simulink model "CDR_240702"  (R2019b)
settings: Solver=ode4  StartTime=0.0  StopTime=inf  FixedStep=BKIN_STEP_TIME  RelTol=1e-3  EnableMultiTasking=on
StartFcn:
  |  warndlg('Dexterit-E models cannot run under simulation. Please compile your model and run it from within Dexterit-E.');set_param(bdroot,'SimulationCommand','stop')
model workspace (MAT data in the model file):
  BKIN_KINEMATIC_FRAME_SIZE = 400
  BKIN_STEP_TIME = 0.00025
  COHERENCY = 9
  CONST_A = 1
  CONST_B = 2
  CONST_C = 3
  CONST_D = 4
  DIRECTION = 10
  DOT_AREA_RADIUS = 5
  DOT_DELAY = 4
  DOT_TARGET = 7
  D_REACH_TARG = 4
  D_START_TARG = 2
  E_DOT_ON = 3
  E_D_REACHED = 5
  E_ND_REACHED = 4
  E_NO_EVENT = 0
  E_REACH_ON = 2
  E_START_ON = 1
  E_TIMED_OUT = 7
  E_TOO_SLOW = 6
  E_TRIAL_END = 8
  HEIGHT = 5
  INCREMENT_TRIGGER = 12
  INC_RES = 7
  INIT_COLOR = 7
  LABEL_HEIGHT = 10
  LABEL_TEXT = 9
  LENGTH = 4
  LOAD_1 = 8
  MAX_REACH_TIME = 1
  ND_REACH_TARG = 3
  ND_START_TARG = 1
  NUMBER_OF_DOTS = 6
  PUSH_BACK = 9
  RADIUS_VIS = 3
  RAMP_DURATION = 10
  RESCALE = 8
  SPEED = 11
  STROKE_COLOR = 8
  STROKE_WIDTH = 6
  TIME_OUT = 2
  TIME_OUT_LABEL = 6
  TOO_SLOW_LABEL = 5
  TRIAL_DELAY = 3
  col_x = 1
  col_y = 2
undefined symbols (not defined in the file): slselsubs
libraries: Video x8, KINARM_EP_loads x5, General x3, KINARM_general x3, slrtlib x2
settings Model: ModifiedComment=chris -- Wed Feb 16 09:18:30 2005 -- Version 1.1384  ModifiedHistory=Feb 16/05 - Add error repeat, add offset ramp  ExtModeArmWhenConnect=off  ExtModeLogAll=off  OrderedModelArguments=off  Creator=Chris Grebeldinger  LastModifiedBy=User
settings SolverCC: AutoInsertRateTranBlk=on
settings DataIOCC: SaveFormat=Array  SignalLoggingSaveFormat=ModelDataLogs  SaveOutput=off  SaveTime=off  ReturnWorkspaceOutputs=off  SignalLoggingName=sigsOut
settings OptimizationCC: BlockReduction=off  BooleanDataType=off  OptimizeBlockIOStorage=off  BufferReuse=off  GlobalBufferReuse=off  ExpressionFolding=off  ExpressionDepthLimit=2147483647  LocalBlockOutputs=off  InitFltsAndDblsToZero=on  LifeSpan=inf  OptimizeDataStoreBuffers=off  BusAssignmentInplaceUpdate=off
settings DebuggingCC: SaveWithParameterizedLinksMsg=none  UnderspecifiedInitializationDetection=Classic  MergeDetectMultiDrivingBlocksExec=none  SignalResolutionControl=TryResolveAllWithWarning  MultiTaskDSMMsg=warning  FcnCallInpInsideContextMsg=warning  BusObjectLabelMismatch=none  StateNameClashWarn=warning  StrictBusMsg=ErrorOnBusTreatedAsVector  SFUnexpectedBacktrackingDiag=warning  SFNoUnconditionalDefaultTransitionDiag=warning  SFExecutionAtInitializationDiag=none  ArithmeticOperatorsInVariantConditions=warning
settings HardwareCC: ProdBitPerPointer=32  ProdBitPerSizeT=32  ProdBitPerPtrDiffT=32  ProdLargestAtomicFloat=None  ProdWordSize=32  ProdLongLongMode=on  ProdHWDeviceType=Generic->32-bit x86 compatible  TargetHWDeviceType=32-bit Generic
settings ModelReferenceCC: PropagateSignalLabelsOutOfModel=off
settings SFSimCC: SimCustomHeaderCode="#include \"stdlib.h\""  SFSimEcho=off  SimUseLocalCustomCode=off  SimParseCustomCode=off  CustomCodeUndefinedFunction=UseInterfaceOnly
settings RTWCC: Description=Simulink Real-Time  SystemTargetFile=slrt.tlc  TemplateMakefile=slrt_default_tmf  RTWUseLocalCustomCode=off  CustomSourceCode="#include \"stdlib.h\""  CodeExecutionProfiling=on  RTWCompilerOptimization=on
settings CodeAppCC: MaxIdLength=63  StateflowObjectComments=on
settings SimulinkRealTimeCC: TargetFcnLib=ansi_tfl_tmw.mat  GeneratePreprocessorConditionals=Disable all  PreserveStateflowLocalDataDimensions=off
settings ConfigComp: CovMetricSettings=dw  CovHtmlReporting=on  CovSaveCumulativeToWorkspaceVar=on  CovSaveSingleToWorkspaceVar=on  CovExternalEMLEnable=off

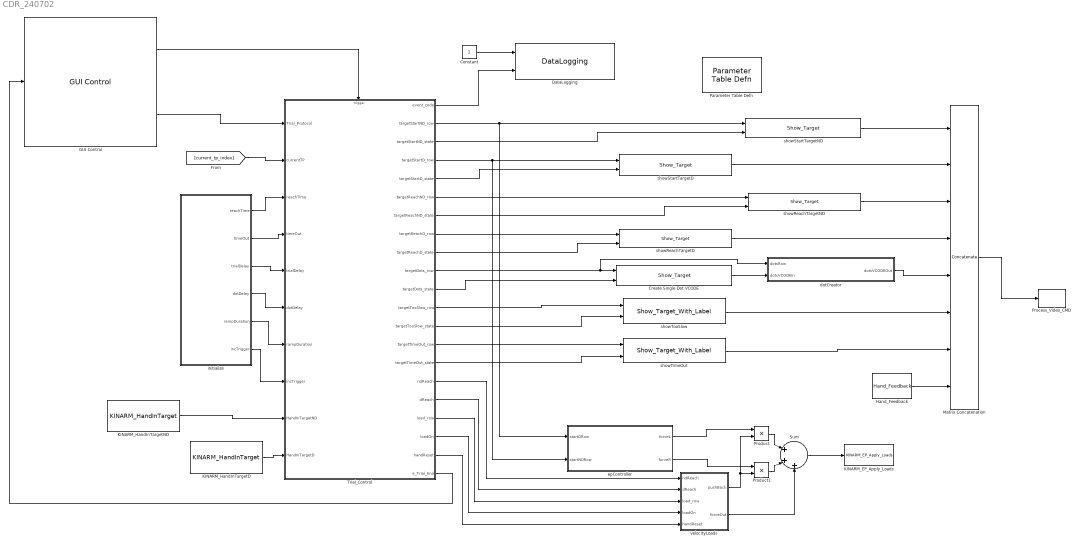
== system CDR_240702 ==
  Constant : Constant
  Create Single Dot VCODE : Video/Show_Target  target_type=Circle  num_states=1  attribcol1=[INIT_COLOR 0 0 RADIUS_VIS]  attribcol2=[0 0 0 0]  attribcol3=[0 0 0 0]  attribcol4=[0 0 0 0]  attribcol5=[0 0 0 0]  stateindices_padding=[0 0 0 0 0 0 0;0 0 0 0 0 0 0;0 0 0 0 0 0 0;0 0 0 0 0 0 0;0 0 0 0 0 0 0]  source=dialog  opacity=100  target_display=Both subject and operator displays  num_col=4
  DataLogging : General/DataLogging  log_event_codes=on  log_analog_inputs=off  show_time_remaining=off  ecat_include=on
  GUI Control : General/GUI Control  task_version=1.0  show_repeat_trial_flag=off  use_custom_tp=off  target_type_str=Circle  Target_Type=1  XYcols=[1 2]  Vcols=3  Lcols=4  indices_padding=[0 0 0 0;0 0 0 0]  target_table_rows=64  load_table_rows=20  tp_table_rows=100
  Hand_Feedback : KINARM_general/Hand_Feedback  feedback_cntl_src=none
  KINARM_EP_Apply_Loads : KINARM_EP_loads/KINARM_EP_Apply_Loads  up_duration=100  down_duration=100  max_force=15
  KINARM_HandInTargetD : KINARM_general/KINARM_HandInTarget  use_dominant_hand=on  target_type=Rectangle  num_states=1  attribcol1=[ LENGTH HEIGHT 0]  attribcol2=[0 0 0]  attribcol3=[0 0 0]  attribcol4=[0 0 0]  attribcol5=[0 0 0]
  KINARM_HandInTargetND : KINARM_general/KINARM_HandInTarget  use_dominant_hand=off  target_type=Rectangle  num_states=1  attribcol1=[ LENGTH HEIGHT 0]  attribcol2=[0 0 0]  attribcol3=[0 0 0]  attribcol4=[0 0 0]  attribcol5=[0 0 0]
  Matrix Concatenation : Concatenate  NumInputs=8  Mode=Multidimensional array
  Parameter Table Defn : General/Parameter Table Defn  ShowInLibBrowser=0
  Process_Video_CMD : Video/Process_Video_CMD  video_delay=0
  Product : Product
  Product1 : Product
  Sum : Sum  Inputs=|+++
  Trial_Control : Stateflow chart  TreatAsAtomicUnit=on
  dotCreator : Subsystem
  epController : Subsystem
  initialize : Subsystem
  showReachTargetD : Video/Show_Target  target_type=Rectangle  num_states=1  attribcol1=[INIT_COLOR STROKE_COLOR STROKE_WIDTH LENGTH HEIGHT 0]  attribcol2=[0 0 0 0 0 0]  attribcol3=[0 0 0 0 0 0]  attribcol4=[0 0 0 0 0 0]  attribcol5=[0 0 0 0 0 0]  stateindices_padding=[0 0 0 0 0;0 0 0 0 0;0 0 0 0 0;0 0 0 0 0;0 0 0 0 0]  source=dialog  opacity=100  target_display=Both subject and operator displays  num_col=6
  showReachTargetND : Video/Show_Target  target_type=Rectangle  num_states=1  attribcol1=[INIT_COLOR STROKE_COLOR STROKE_WIDTH LENGTH HEIGHT 0]  attribcol2=[0 0 0 0 0 0]  attribcol3=[0 0 0 0 0 0]  attribcol4=[0 0 0 0 0 0]  attribcol5=[0 0 0 0 0 0]  stateindices_padding=[0 0 0 0 0;0 0 0 0 0;0 0 0 0 0;0 0 0 0 0;0 0 0 0 0]  source=dialog  opacity=100  target_display=Both subject and operator displays  num_col=6
  showStartTargetD : Video/Show_Target  target_type=Rectangle  num_states=1  attribcol1=[INIT_COLOR STROKE_COLOR STROKE_WIDTH LENGTH HEIGHT 0]  attribcol2=[0 0 0 0 0 0]  attribcol3=[0 0 0 0 0 0]  attribcol4=[0 0 0 0 0 0]  attribcol5=[0 0 0 0 0 0]  stateindices_padding=[0 0 0 0 0;0 0 0 0 0;0 0 0 0 0;0 0 0 0 0;0 0 0 0 0]  source=dialog  opacity=100  target_display=Both subject and operator displays  num_col=6
  showStartTargetND : Video/Show_Target  target_type=Rectangle  num_states=1  attribcol1=[INIT_COLOR STROKE_COLOR STROKE_WIDTH LENGTH HEIGHT 0]  attribcol2=[0 0 0 0 0 0]  attribcol3=[0 0 0 0 0 0]  attribcol4=[0 0 0 0 0 0]  attribcol5=[0 0 0 0 0 0]  stateindices_padding=[0 0 0 0 0;0 0 0 0 0;0 0 0 0 0;0 0 0 0 0;0 0 0 0 0]  source=dialog  opacity=100  target_display=Both subject and operator displays  num_col=6
  showTimeOut : Video/Show_Target_With_Label  target_type=Circle  num_states=1  attribcol1=[0 0 0 0 LABEL_TEXT INIT_COLOR LABEL_HEIGHT]  attribcol2=[0 0 0 0 0 0 0]  attribcol3=[0 0 0 0 0 0 0]  attribcol4=[0 0 0 0 0 0 0]  attribcol5=[0 0 0 0 0 0 0]  stateindices_padding=[0 0 0 0;0 0 0 0;0 0 0 0;0 0 0 0;0 0 0 0]  source=dialog  opacity=100  target_display=Both subject and operator displays
  showTooSlow : Video/Show_Target_With_Label  target_type=Circle  num_states=1  attribcol1=[0 0 0 0 LABEL_TEXT INIT_COLOR LABEL_HEIGHT]  attribcol2=[0 0 0 0 0 0 0]  attribcol3=[0 0 0 0 0 0 0]  attribcol4=[0 0 0 0 0 0 0]  attribcol5=[0 0 0 0 0 0 0]  stateindices_padding=[0 0 0 0;0 0 0 0;0 0 0 0;0 0 0 0;0 0 0 0]  source=dialog  opacity=100  target_display=Both subject and operator displays
  velocityLoads : Subsystem
  wires:
  KINARM_HandInTargetND/1 -> Trial_Control/9(HandInTargetND)
  GUI Control/2 -> Trial_Control/1(Trial_Protocol)
  Trial_Control/21(e_Trial_End) -> GUI Control/1
  GUI Control/1 -> Trial_Control/Trigger
  Trial_Control/7(targetReachND_state) -> showReachTargetND/2
  Trial_Control/6(targetReachND_row) -> showReachTargetND/1
  Matrix Concatenation/1 -> Process_Video_CMD/1
  Hand_Feedback/1 -> Matrix Concatenation/8
  Trial_Control/8(targetReachD_row) -> showReachTargetD/1
  Trial_Control/9(targetReachD_state) -> showReachTargetD/2
  Trial_Control/1(event_code) -> DataLogging/2
  Constant/1 -> DataLogging/1
  KINARM_HandInTargetD/1 -> Trial_Control/10(HandInTargetD)
  initialize/1(reachTime) -> Trial_Control/3(reachTime)
  initialize/2(timeOut) -> Trial_Control/4(timeOut)
  Trial_Control/11(targetDots_state) -> Create Single Dot VCODE/2
  Create Single Dot VCODE/1 -> dotCreator/2(dotsVCODEIn)
  Trial_Control/10(targetDots_row) -> dotCreator/1(dotsRow), Create Single Dot VCODE/1
  dotCreator/1(dotsVCODEOut) -> Matrix Concatenation/5
  showReachTargetND/1 -> Matrix Concatenation/3
  showReachTargetD/1 -> Matrix Concatenation/4
  showStartTargetD/1 -> Matrix Concatenation/2
  showStartTargetND/1 -> Matrix Concatenation/1
  initialize/3(trialDelay) -> Trial_Control/5(trialDelay)
  Trial_Control/2(targetStartND_row) -> epController/1(startDRow), showStartTargetND/1
  Trial_Control/5(targetStartD_state) -> showStartTargetD/2
  initialize/4(dotDelay) -> Trial_Control/6(dotDelay)
  [current_tp_index] -> Trial_Control/2(currentTP)
  Trial_Control/3(targetStartND_state) -> showStartTargetND/2
  Trial_Control/4(targetStartD_row) -> showStartTargetD/1, epController/2(startNDRow)
  Trial_Control/18(load_row) -> velocityLoads/3(load_row)
  Trial_Control/16(ndReach) -> velocityLoads/1(ndReach)
  Trial_Control/17(dReach) -> velocityLoads/2(dReach)
  Trial_Control/19(loadOn) -> velocityLoads/4(loadOn)
  Sum/1 -> KINARM_EP_Apply_Loads/1
  velocityLoads/2(forceOut) -> Sum/3
  Product1/1 -> Sum/2
  Product/1 -> Sum/1
  Trial_Control/20(handReset) -> velocityLoads/5(handReset)
  epController/1(forceL) -> Product/1
  epController/2(forceR) -> Product1/1
  initialize/6(incTrigger) -> Trial_Control/8(incTrigger)
  Trial_Control/12(targetTooSlow_row) -> showTooSlow/1
  Trial_Control/13(targetTooSlow_state) -> showTooSlow/2
  Trial_Control/15(targetTimeOut_state) -> showTimeOut/2
  Trial_Control/14(targetTimeOut_row) -> showTimeOut/1
  showTimeOut/1 -> Matrix Concatenation/7
  showTooSlow/1 -> Matrix Concatenation/6
  velocityLoads/1(pushBack) -> Product/2, Product1/2
  initialize/5(rampDuration) -> Trial_Control/7(rampDuration)

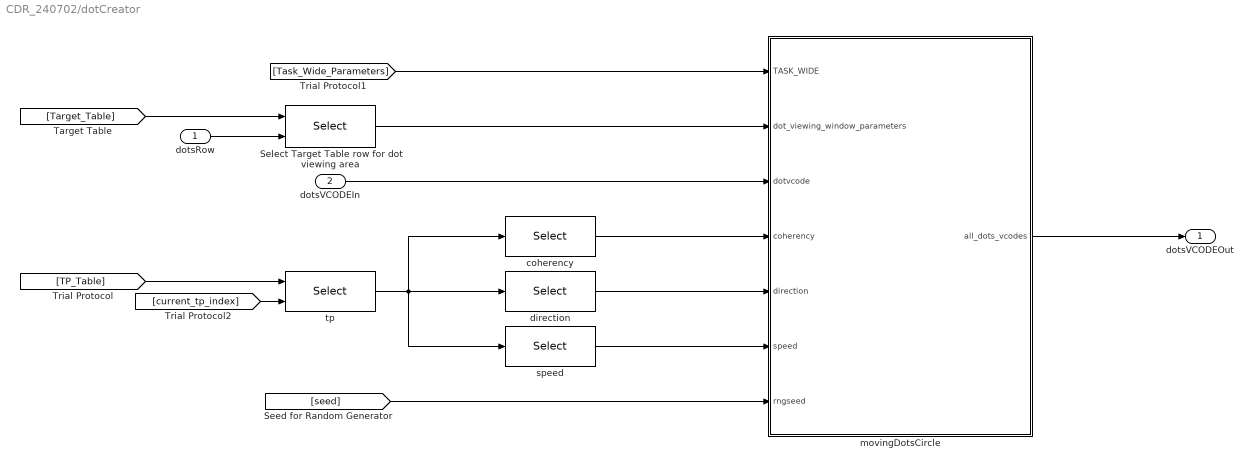
== system CDR_240702/dotCreator ==
  dotsRow : Inport
  dotsVCODEIn : Inport  Port=2
  Select Target Table row for dot viewing area : Selector  NumberOfDimensions=2  IndexOptions=Index vector (port),Index vector (dialog)  Indices=[SPEED],[col_x col_y]  OutputSizes=1,1
  coherency : Selector  IndexOptions=Index vector (dialog)  Indices=[COHERENCY]  OutputSizes=1
  direction : Selector  IndexOptions=Index vector (dialog)  Indices=[DIRECTION]  OutputSizes=1
  movingDotsCircle : MATLAB Function  TreatAsAtomicUnit=on  SystemSampleTime=0.02
  speed : Selector  IndexOptions=Index vector (dialog)  Indices=[SPEED]  OutputSizes=1
  tp : Selector  NumberOfDimensions=2  IndexOptions=Index vector (port),Select all  Indices=[COHERENCY],100  OutputSizes=1,100
  dotsVCODEOut : Outport
  wires:
  movingDotsCircle/1(all_dots_vcodes) -> dotsVCODEOut/1
  Select Target Table row for dot viewing area/1 -> movingDotsCircle/2(dot_viewing_window_parameters)
  coherency/1 -> movingDotsCircle/4(coherency)
  direction/1 -> movingDotsCircle/5(direction)
  speed/1 -> movingDotsCircle/6(speed)
  [seed] -> movingDotsCircle/7(rngseed)
  [Target_Table] -> Select Target Table row for dot viewing area/1
  dotsVCODEIn/1 -> movingDotsCircle/3(dotvcode)
  dotsRow/1 -> Select Target Table row for dot viewing area/2
  [Task_Wide_Parameters] -> movingDotsCircle/1(TASK_WIDE)
  [TP_Table] -> tp/1
  [current_tp_index] -> tp/2
  tp/1 -> direction/1, speed/1, coherency/1

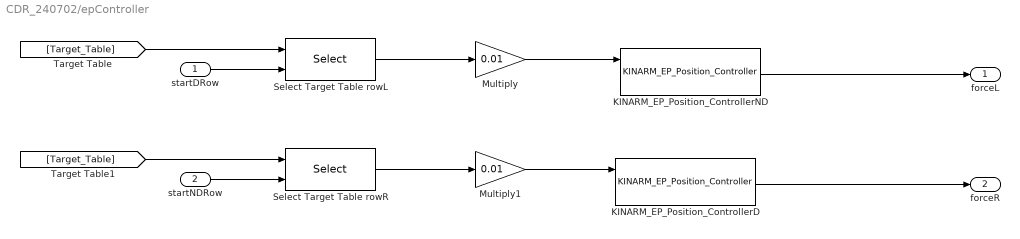
== system CDR_240702/epController ==
  startDRow : Inport
  startNDRow : Inport  Port=2
  KINARM_EP_Position_ControllerD : KINARM_EP_loads/KINARM_EP_Position_Controller  use_dom_hand=on  inertias_for_FF=KINARM End Point robot  gain_choice=Standard Movement  sample_time=0.001
  KINARM_EP_Position_ControllerND : KINARM_EP_loads/KINARM_EP_Position_Controller  use_dom_hand=off  inertias_for_FF=KINARM End Point robot  gain_choice=Standard Movement  sample_time=0.001
  Multiply : Gain  Gain=0.01
  Multiply1 : Gain  Gain=0.01
  Select Target Table rowL : Selector  NumberOfDimensions=2  IndexOptions=Index vector (port),Index vector (dialog)  Indices=[SPEED],[col_x col_y]  OutputSizes=1,1
  Select Target Table rowR : Selector  NumberOfDimensions=2  IndexOptions=Index vector (port),Index vector (dialog)  Indices=[SPEED],[col_x col_y]  OutputSizes=1,1
  forceL : Outport
  forceR : Outport  Port=2
  wires:
  [Target_Table] -> Select Target Table rowL/1
  startDRow/1 -> Select Target Table rowL/2
  startNDRow/1 -> Select Target Table rowR/2
  [Target_Table] -> Select Target Table rowR/1
  Select Target Table rowR/1 -> Multiply1/1
  KINARM_EP_Position_ControllerND/1 -> forceL/1
  Select Target Table rowL/1 -> Multiply/1
  Multiply/1 -> KINARM_EP_Position_ControllerND/1
  Multiply1/1 -> KINARM_EP_Position_ControllerD/1
  KINARM_EP_Position_ControllerD/1 -> forceR/1

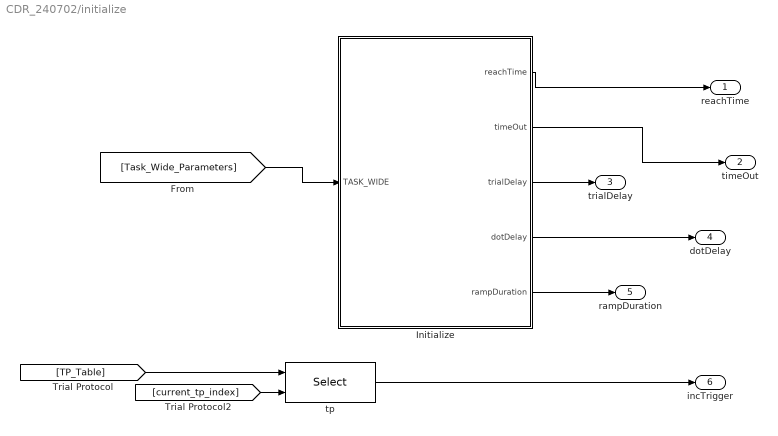
== system CDR_240702/initialize ==
  Initialize : MATLAB Function  TreatAsAtomicUnit=on
  tp : Selector  NumberOfDimensions=2  IndexOptions=Index vector (port),Index vector (dialog)  Indices=[COHERENCY],[INCREMENT_TRIGGER]  OutputSizes=1,100
  reachTime : Outport
  timeOut : Outport  Port=2
  trialDelay : Outport  Port=3
  dotDelay : Outport  Port=4
  rampDuration : Outport  Port=5
  incTrigger : Outport  Port=6
  wires:
  Initialize/1(reachTime) -> reachTime/1
  [Task_Wide_Parameters] -> Initialize/1(TASK_WIDE)
  Initialize/2(timeOut) -> timeOut/1
  Initialize/3(trialDelay) -> trialDelay/1
  Initialize/4(dotDelay) -> dotDelay/1
  tp/1 -> incTrigger/1
  [current_tp_index] -> tp/2
  [TP_Table] -> tp/1
  Initialize/5(rampDuration) -> rampDuration/1

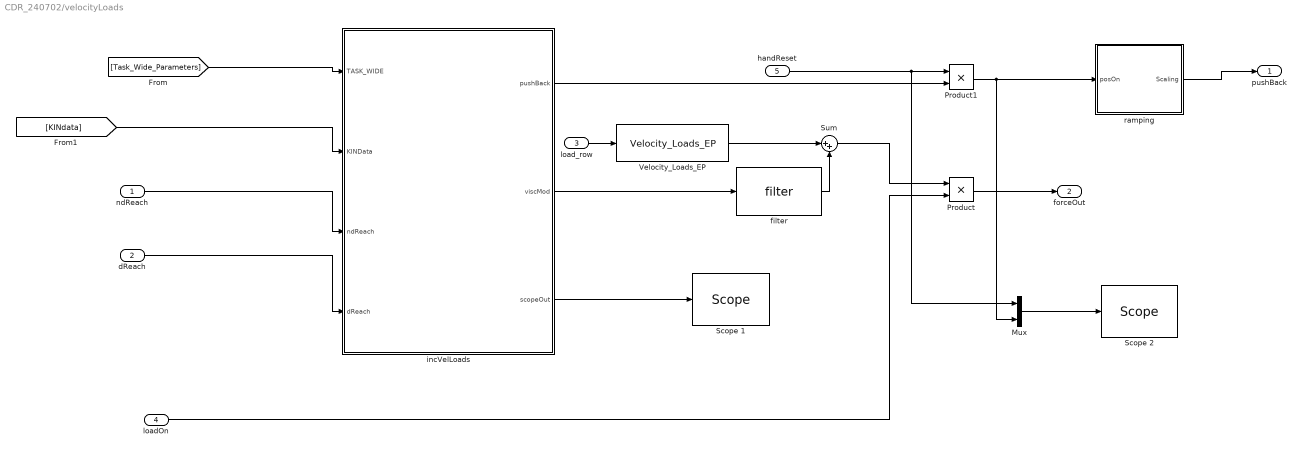
== system CDR_240702/velocityLoads ==
  ndReach : Inport
  dReach : Inport  Port=2
  load_row : Inport  Port=3
  loadOn : Inport  Port=4
  handReset : Inport  Port=5
  Mux : Mux  Inputs=2
  Product : Product
  Product1 : Product
  Scope 1 : slrtlib/Displays and Logging/Scope   scopeno=1  scopetype=Target  autostart=on  viewmode=Numerical  formatstr='%15.6f'  grid=on  ylimits=[0,0]  nosamples=250  noprepostsamples=0  interleave=1  triggermode=FreeRun  triggersignal=1  trigsignalfromport=off  triggerlevel=0.0  triggerslope=Either  triggerscope=1  triggersample=0  filename=data.dat  mode=Lazy  writesize=512  autorestart=off  dynamicfilemode=off  maxwritefilesize=512*1024^2
  Scope 2 : slrtlib/Displays and Logging/Scope   scopeno=2  scopetype=Target  autostart=on  viewmode=Numerical  formatstr='%15.6f'  grid=on  ylimits=[0,0]  nosamples=250  noprepostsamples=0  interleave=1  triggermode=FreeRun  triggersignal=1  trigsignalfromport=off  triggerlevel=0.0  triggerslope=Either  triggerscope=1  triggersample=0  filename=data.dat  mode=Lazy  writesize=512  autorestart=off  dynamicfilemode=off  maxwritefilesize=512*1024^2
  Sum : Sum  Inputs=|++
  Velocity_Loads_EP : KINARM_EP_loads/Velocity_Loads_EP  use_dom_hand=on  loadcol=[1 2 3 4]  source=dialog  scaling=1  stability=on
  filter : KINARM_EP_loads/Velocity_Loads_EP/filter  SystemSampleTime=-1  Latency=0  AutoFrameSizeCalculation=off
  incVelLoads : MATLAB Function  TreatAsAtomicUnit=on  SystemSampleTime=0.02
  ramping : Subsystem  mask(Perturbation){}
  pushBack : Outport
  forceOut : Outport  Port=2
  wires:
  [Task_Wide_Parameters] -> incVelLoads/1(TASK_WIDE)
  incVelLoads/2(viscMod) -> filter/1
  Product/1 -> forceOut/1
  loadOn/1 -> Product/2
  load_row/1 -> Velocity_Loads_EP/1
  ndReach/1 -> incVelLoads/3(ndReach)
  dReach/1 -> incVelLoads/4(dReach)
  Velocity_Loads_EP/1 -> Sum/1
  incVelLoads/3(scopeOut) -> Scope 1/1
  incVelLoads/1(pushBack) -> Product1/2
  handReset/1 -> Mux/1, Product1/1
  Product1/1 -> ramping/1(posOn), Mux/2
  [KINdata] -> incVelLoads/2(KINData)
  Sum/1 -> Product/1
  filter/1 -> Sum/2
  Mux/1 -> Scope 2/1
  ramping/1(Scaling) -> pushBack/1

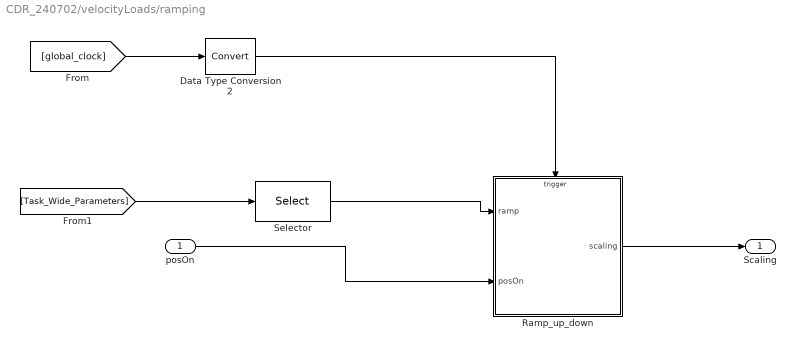
== system CDR_240702/velocityLoads/ramping ==
  posOn : Inport
  Data Type Conversion2 : DataTypeConversion
  Ramp_up_down : Stateflow chart  TreatAsAtomicUnit=on
  Selector : Selector  NumberOfDimensions=2  InputPortWidth=3  IndexOptions=Index vector (dialog),Select all  Indices=[RAMP_DURATION],[3]  OutputSizes=slselsubs([(-2),(-2)],1),1
  Scaling : Outport
  wires:
  Ramp_up_down/1(scaling) -> Scaling/1
  [global_clock] -> Data Type Conversion2/1
  Data Type Conversion2/1 -> Ramp_up_down/Trigger
  [Task_Wide_Parameters] -> Selector/1
  Selector/1 -> Ramp_up_down/1(ramp)
  posOn/1 -> Ramp_up_down/2(posOn)

== stateflow chart CDR_240702/Trial_Control ==
  settings: sampleTime=0.001
  state MainTrial
    state showReach/
      entry:
      event_code = E_REACH_ON;
      targetReachND_state = 1;
      targetReachD_state = 1;
    state showStartTargets/
      entry:
      event_code = E_START_ON;
      targetStartND_state = 1;
      targetStartD_state = 1;
      handReset = 0;
      loadOn = 0;
    state showDots/
      entry:
      loadOn = 1;
      event_code = E_DOT_ON;
      targetDots_state = 1;
    state leftReached/
      entry:
      event_code = E_D_REACHED;
      dReach = dReach + 1;
    state rightReached/
      entry:
      event_code = E_ND_REACHED;
      ndReach = ndReach + 1;
    state noIncrement/
      entry:
      ndReach = 0;
      dReach = 0;
    state tooSlow/
      % Set the post-trial delay.
      entry:
      event_code = E_TOO_SLOW;
      targetTooSlow_state = 1;
      targetDots_state = 0;
    state timedOut/
      % Set the post-trial delay.
      entry:
      event_code = E_TIMED_OUT;
      targetTimeOut_state = 1;
      targetDots_state = 0;
    state statesOff/
      entry:
      targetDots_state = 0;
      targetReachND_state = 0;
      targetReachD_state = 0;
      targetStartND_state = 0;
      targetStartD_state = 0;
      loadOn = 0;
      handReset = 1;
    state EndOfTrial/
      % Set the post-trial delay.
      entry:
      targetTooSlow_state = 0;
      targetTimeOut_state = 0;
      event_code = E_TRIAL_END;
    showStartTargets -> timedOut [order 2] : after(timeOut, msec)
    showStartTargets -> showReach [order 1] : [HandInTargetD(targetStartD_row) == 1 && HandInTargetND(targetStartND_row) == 1]
    showReach -> showStartTargets [order 1] : [HandInTargetD(targetStartD_row) == 0]
    showReach -> showStartTargets [order 2] : [HandInTargetND(targetStartND_row) == 0]
    showReach -> showDots [order 3] : after(dotDelay,msec)
    showDots -> leftReached [order 3] : [HandInTargetD(targetReachD_row) == 1]
    showDots -> rightReached [order 2] : [HandInTargetND(targetReachND_row) == 1]
    leftReached -> (junction 76)
    showDots -> tooSlow [order 1] : after(reachTime, msec)
    rightReached -> (junction 76)
    (junction 76) -> noIncrement [order 2] : [incTrigger == 0]
    (junction 76) -> statesOff [order 1] : after(trialDelay, msec)
    noIncrement -> statesOff : after(trialDelay, msec)
    tooSlow -> EndOfTrial : after(trialDelay*4,msec)
    timedOut -> EndOfTrial : after(trialDelay*4,msec)
    statesOff -> EndOfTrial : after(rampDuration, msec)
  state Initialize/
    entry:
    targetDots_row = Trial_Protocol(DOT_TARGET);
    load_row = Trial_Protocol(LOAD_1);
    targetDots_state = 0;
    targetStartND_row = Trial_Protocol(ND_START_TARG);
    targetStartND_state = 0;
    targetStartD_row = Trial_Protocol(D_START_TARG);
    targetStartD_state = 0;
    targetReachND_row = Trial_Protocol(ND_REACH_TARG);
    targetReachND_state = 0;
    targetReachD_row = Trial_Protocol(D_REACH_TARG);
    targetReachD_state = 0;
    targetTooSlow_row = Trial_Protocol(TOO_SLOW_LABEL);
    targetTooSlow_state = 0;
    targetTimeOut_row = Trial_Protocol(TIME_OUT_LABEL);
    targetTimeOut_state = 0;
    ndReach = 0;
    dReach = 0;
  state Inter_Trial_State/
    entry:
    event_code = 0;
    targetDots_state = 0;
    targetReachND_state = 0;
    targetReachD_state = 0;
    targetStartND_state = 0;
    targetStartD_state = 0;
    targetTooSlow_state = 0;
    targetTimeOut_state = 0;
    handReset = 0;
    loadOn = 0;
    e_Trial_End;
  (default) -> Initialize
  Initialize -> showStartTargets : [currentTP > 0]
  Inter_Trial_State -> showStartTargets : after(1, msec)
  MainTrial -> Inter_Trial_State : e_ExitTrialNow
  EndOfTrial -> Inter_Trial_State : after(rampDuration*2,msec)
  data: Trial_Protocol input double; currentTP input; event_code output [0..] =0; targetStartND_row output; targetStartND_state output; targetStartD_row output; targetStartD_state output; targetReachND_row output [1..32]; targetReachND_state output double; targetReachD_row output double; targetReachD_state output double; targetDots_row output; targetDots_state output; targetTooSlow_row output; targetTooSlow_state output; targetTimeOut_row output; targetTimeOut_state output; reachTime input; timeOut input; trialDelay input; dotDelay input; rampDuration input; incTrigger input; HandInTargetND input double; HandInTargetD input; ndReach output; dReach output; load_row output; loadOn output; handReset output
  data targetReachND_row settings: description=index of the row currently being used in the TargetTable
  events: e_clk input RISING_EDGE_EVENT; e_ExitTrialNow input EITHER_EDGE_EVENT; e_Trial_End output EITHER_EDGE_EVENT

== matlab function CDR_240702/dotCreator/movingDotsCircle ==
  data: TASK_WIDE input; dot_viewing_window_parameters input; dotvcode input; all_dots_vcodes output; coherency input; direction input; speed input; rngseed input; NUMBER_OF_DOTS parameter; DOT_AREA_RADIUS parameter; BKIN_STEP_TIME parameter; RESCALE parameter
function all_dots_vcodes   = build_dot_vcodes(TASK_WIDE, dot_viewing_window_parameters, dotvcode, coherency, direction, speed, rngseed, NUMBER_OF_DOTS, DOT_AREA_RADIUS, BKIN_STEP_TIME, RESCALE)
% This function will generate the vcodes for all dots.
% Defn: signal dots are dots moving coherently with same speed in same
%       direction
% Defn: noise dots are dots moving in a random direction with a random
%       speed
%
% inputs - dotvcode, the vcode for a single dot
%        - coherency, the fraction of dots that are signal dots      
%        - the direction of movement for the signal dots (+ve is
%        right, -ve is left)
%        - number_of_dots, the total number of dots to be displaying
%        - dot_viewing_window_parameters, the x and y position of the
%        viewing area and its length
%        - speed of the signal dots (cm/s). The noise dots will be moving at 
%          a speed that is anywhere from 50% slower to 150% faster than 
%          this speed
%        - rngseed, a seed for the random number generator
% output - updated_dots_vcode, these are the vcodes that will draw the dots

%random dot generator modified by Kayne Park 2024 to display random dots in
%a circle rather than rectangle

MAX_VCODES = 40; % number of vcodes reserved for the dots
MAX_REPEATS = 25; % the maximum number of targets displayed per vcode
MAX_NUM_DOTS = MAX_VCODES * MAX_REPEATS; % the max number of dots we can have
BLOCK_SAMPLE_TIME = BKIN_STEP_TIME;    % THIS MUST MATCH THE SAMPLE TIME OF THE BLOCK

reScale = TASK_WIDE(RESCALE)/100;
dotAreaRadius = TASK_WIDE(DOT_AREA_RADIUS)/100;
number_of_dots = TASK_WIDE(NUMBER_OF_DOTS);

% The centre of the dot viewing window
x0 = dot_viewing_window_parameters(1)/100;
y0 = dot_viewing_window_parameters(2)/100;

persistent X Y init; % here we store the x and y positions of all our dots

if isempty(X)
    X = zeros(1, MAX_NUM_DOTS);
    Y = zeros(1, MAX_NUM_DOTS);
    
    init = 0;
end   

% Check if the dot vcode status is set to draw
% If not, do nothing
if dotvcode(2) == 0
    all_dots_vcodes = zeros(MAX_VCODES, 70);
    
    init = 0;
else
    num_signal_dots = floor(coherency * number_of_dots); % calculate the number of signal dots
    num_noise_dots = number_of_dots - num_signal_dots; % calculate the number of noise dots
    
    % Initializing the vcodes for all dots 
    all_dots_vcodes = zeros(MAX_VCODES, 70);
    
    % All the vcodes in all_dots_vcodes have the same settings except all_dots_vcodes(16), which sets the
    % number of dots to show for that vcode and all_dots_vcodes(17:66) which are the position(s) of the dots
    % This loop sets all parameters except for position(s).
    for ii  = 1:ceil(number_of_dots/MAX_REPEATS)
        all_dots_vcodes(1:MAX_VCODES,1) = dotvcode(1) + 20; % set the shape to be repeated
        all_dots_vcodes(ii,2:end) = dotvcode(2:end); % set the rest of the vcode specifications
        % let each vcode know how many repeats that vcode has (except the
        % last row, which happens after the loop)
        all_dots_vcodes(ii, 16) = MAX_REPEATS;
    end
    % Set the correct amount of dots for the last vcode
    all_dots_vcodes(ceil(number_of_dots/MAX_REPEATS),16) = rem(number_of_dots,MAX_REPEATS);           

    % Generate starting locations for dots if the dots were just turned
    % on
    % Even though we do not need X and Y to be of size MAX_NUM_DOTS, we set
    % the size of X and Y to MAX_NUM_DOTS because this makes the subsequent
    % positioning code simpler. 
    if init == 0
        rng(rngseed)                
        t = 2*pi*rand(1, MAX_NUM_DOTS);
        r = dotAreaRadius*sqrt(rand(1, MAX_NUM_DOTS));
        X = x0 + r.*cos(t); % x coordinates for a circle      
        Y = y0 + r.*sin(t); % y coordinates
        
        init = 1;
    end

    % Compiled code requires an upper limit (i.e. static vector size) so
    % the noise_dots and signal_dots vectors need to have a initial size of
    % MAX_NUM_DOTS. We then only use a subset of each of those vectors.
    
    % Each time step, identify a new sub-set of dots that will be noise
    % dots (i.e. whether a dot is a noise or not changes each time-step)
    % Note: during compilation, randperm() requires the output size to be
    % fixed, so we cannot call randperm(number_of_dots). The following code
    % is equivalent to randperm(number_of_dots, num_noise_dots).
    noise_dots = randperm(MAX_NUM_DOTS); 
    noise_dots = noise_dots(noise_dots < number_of_dots+1);
    noise_dots = noise_dots(1:num_noise_dots); % set of indexes that correspond to the noise dots

    % Then all the dots that aren't noise dots are set to signal dots
    signal_dots = 1:MAX_NUM_DOTS;
    signal_dots = signal_dots(signal_dots < number_of_dots+1);
    signal_dots(noise_dots) = []; % set of all indeces that correspond to the signal dots
        
    % We now move the dots!

    % Calculate signal_dot_speed (i.e. the speed of the signal dots)   
    % The units of 'speed' are [cm/s] while signal_dot_speed has to be [m/BLOCK_SAMPLE_TIME]
    signal_dot_speed = BLOCK_SAMPLE_TIME*speed; 
    
    % Calculate the new speed and direction of noise dots. The random speeds assigned to each 
    % noise dot is anywhere from 0.5*signal_dot_speed to 1.5*signal_dot_speed  
    theta = 2*pi*rand(1,length(noise_dots)); % random direction of propagation      
    noise_dot_speed = signal_dot_speed*(rand(1,length(noise_dots))+0.5);
    
    % Calculate the new positions of signal dots based on their velocity
    % (these dots do not move in the y direction)
    X(signal_dots) = X(signal_dots) + direction.*signal_dot_speed; % again, direction is +ve for right, -ve for left
    
    % Calculate the new positions of noise dots based on their individual
    % speed and direction
    X(noise_dots) = X(noise_dots) + noise_dot_speed.*cos(theta); % updating the noise dots' x position
    Y(noise_dots) = Y(noise_dots) + noise_dot_speed.*sin(theta); % updating the noise dots' y position
    
    % Wrap the positions of any dots that have gone out of bounds
    xlimPos = x0+sqrt(dotAreaRadius.^2-(y0-Y).^2);
    xlimNeg = x0-sqrt(dotAreaRadius.^2-(y0-Y).^2);
    ylimPos = y0+sqrt(dotAreaRadius.^2-(x0-X).^2);
    ylimNeg = y0-sqrt(dotAreaRadius.^2-(x0-X).^2);
    
%     X(X < xlimNeg) = X(X < xlimNeg) + sqrt(dotAreaRadius.^2-(y0-Y(X < xlimNeg)).^2)*(2); % dots too far left wrap to the right side
%     Y(Y < ylimNeg) = Y(Y < ylimNeg) + sqrt(dotAreaRadius.^2-(x0-X(Y < ylimNeg)).^2)*(2); % dots under the dot area wrap to the top
%     X(X > xlimPos) = X(X > xlimPos) - sqrt(dotAreaRadius.^2-(y0-Y(X > xlimPos)).^2)*(2); % dots that are too far right wrap to the left side
%     Y(Y > ylimPos) = Y(Y > ylimPos) - sqrt(dotAreaRadius.^2-(x0-X(Y > ylimPos)).^2)*(2); % dots over the top of the dot area wrap to the bottom

    X(((x0-X).^2+(y0-Y).^2)>dotAreaRadius.^2) = x0-((X(((x0-X).^2+(y0-Y).^2)>dotAreaRadius.^2)-x0)*reScale);
    Y(((x0-X).^2+(y0-Y).^2)>dotAreaRadius.^2) = y0-((Y(((x0-X).^2+(y0-Y).^2)>dotAreaRadius.^2)-y0)*reScale);

%     Y(((x0-X).^2+(y0-Y).^2)>dotAreaRadius.^2) = y0-(sign(Y(((x0-X).^2+(y0-Y).^2)>dotAreaRadius.^2)).*abs(abs(y0)-abs(Y(((x0-X).^2+(y0-Y).^2)>dotAreaRadius.^2)))*0.99);

%     Y(((x0-X).^2+(y0-Y).^2)>dotAreaRadius.^2) = ((Y(((x0-X).^2+(y0-Y).^2)>dotAreaRadius.^2))-(sign(Y(((x0-X).^2+(y0-Y).^2)>dotAreaRadius.^2)).*abs(abs(y0)-abs(Y(((x0-X).^2+(y0-Y).^2)>dotAreaRadius.^2)))*0.99));

    % Rearrange the X and Y matrices so that they fit the x, y coordinates in our output vcode           
    all_dots_vcodes(:,17:66) = reshape([X; Y], [2*MAX_REPEATS, MAX_VCODES])';

end

== matlab function CDR_240702/initialize/Initialize ==
  data: TASK_WIDE input; reachTime output; timeOut output; MAX_REACH_TIME parameter; TIME_OUT parameter; trialDelay output; TRIAL_DELAY parameter; dotDelay output; DOT_DELAY parameter; rampDuration output; RAMP_DURATION parameter
function [reachTime, timeOut, trialDelay, dotDelay, rampDuration] = fcn(TASK_WIDE, MAX_REACH_TIME, TIME_OUT, TRIAL_DELAY, DOT_DELAY, RAMP_DURATION)

reachTime = TASK_WIDE(MAX_REACH_TIME);
timeOut = TASK_WIDE(TIME_OUT);
trialDelay = TASK_WIDE(TRIAL_DELAY);
dotDelay = TASK_WIDE(DOT_DELAY);
rampDuration = TASK_WIDE(RAMP_DURATION);

== matlab function CDR_240702/velocityLoads/incVelLoads ==
  data: pushBack output; TASK_WIDE input; KINData input; ndReach input; dReach input; viscMod output; INC_RES parameter; scopeOut output; PUSH_BACK parameter
function [pushBack, viscMod, scopeOut]  = increaseVelLoads(TASK_WIDE, KINData, ndReach, dReach, INC_RES, PUSH_BACK)

incRes = TASK_WIDE(INC_RES);
pushBack = TASK_WIDE(PUSH_BACK);

reachInc = dReach;
if (KINData(3,1) == 2)
    velY = KINData(2,26);
    viscMod = [0,0,0, velY*(incRes*reachInc)];
else
    velY = KINData(1,26);
    viscMod = [0,velY*(incRes*reachInc), 0,0];
end

scopeOut = [viscMod,incRes,reachInc];

== stateflow chart CDR_240702/velocityLoads/ramping/Ramp_up_down ==
  state peak/
    entry:
    scaling=1;
  state RampingUp/
    %sigmoidal ramping taken from Ethan Heming and
    %modified by Kayne
    entry:
    tick=0;
    CurrScale=scaling;
    b=ramp/4; % Center at Middle;
    c=ramp/20; % Define Rise Rate;
    during:
    tick++;
    scaling = (1-CurrScale)/(1+exp(-1*(tick-b)/c))+CurrScale;
  state RampingDown/
    entry:
    tick=0;
    CurrScale=scaling;
    b=ramp/4; % Center at Middle;
    c=ramp/20; % Define Drop Rate;
    during:
    tick++;
    scaling = CurrScale*(1-1/(1+exp(-1*(tick-b)/c)));
  state minimum/
    entry:
    scaling=0;
  peak -> RampingDown : %check if forcefield is turned off
      | [posOn == 0]
  RampingUp -> peak : after(ramp, e_clk)
  RampingDown -> minimum : after(ramp, e_clk)
  minimum -> RampingUp : %check if hand is in target and
      | %trial has a forcefield
      | [posOn == 1]
  (default) -> minimum
  data: ramp input double; scaling output double; tick local double; c local double; b local double; CurrScale local double; posOn input double
  events: e_clk input RISING_EDGE_EVENT
